simulink model "AmplifyFilterDryElectrodesCM"  (R2020b)
settings: Solver=VariableStepAuto  StartTime=0.0  StopTime=27  RelTol=1e-3
libraries: fl_lib x49, ee_lib x11, nesl_utility x6, simulink x2
settings Model: Creator=Miodrag Bolic  LastModifiedBy=bolic

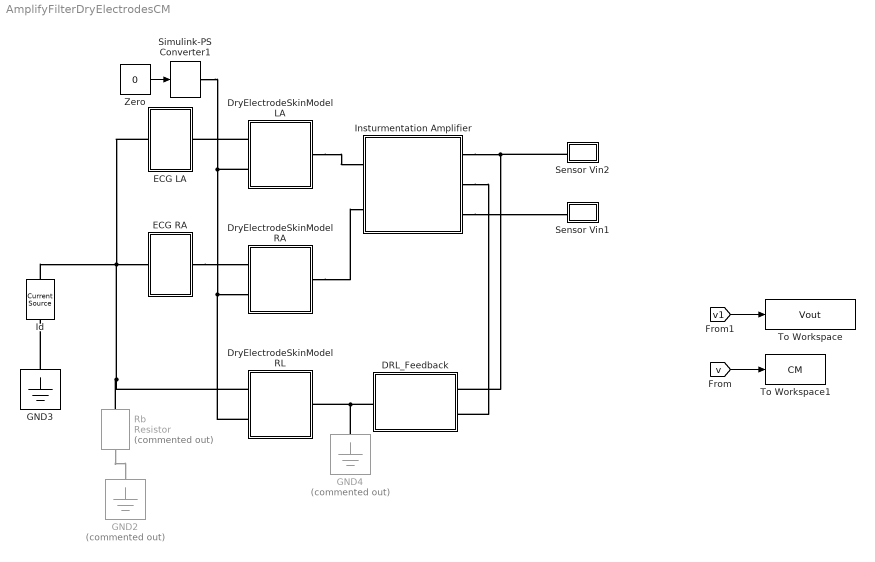
== system AmplifyFilterDryElectrodesCM ==
  DRL_Feedback : Subsystem
  DryElectrodeSkinModelLA : Subsystem
  DryElectrodeSkinModelRA : Subsystem
  DryElectrodeSkinModelRL : Subsystem
  ECG LA : Subsystem
  ECG RA : Subsystem
  GND2 : fl_lib/Electrical/Electrical Elements/Electrical Reference  Commented=on
  GND3 : fl_lib/Electrical/Electrical Elements/Electrical Reference
  GND4 : fl_lib/Electrical/Electrical Elements/Electrical Reference  Commented=on
  Id : ee_lib/Sources/Current Source  dc_current=0.2 uA  ac_current=0.2 uA  ac_shift=0 rad  ac_frequency=60 Hz  noise_mode=0  PSD=0 A^2/Hz  repeatability=1  auto_seed=113289902  user_seed=0  sample_time=1e-3 s  i_specify=off  i_priority=None  i=0 A  i_nominal_specify=off  i_nominal_unit=A  i_nominal_value=1  v_specify=off  v_priority=None  v=0 V  v_nominal_specify=off  v_nominal_unit=V  v_nominal_value=1
      settings: SourceProductBaseCode=PS
  Insturmentation Amplifier : Subsystem
  Rb : fl_lib/Electrical/Electrical Elements/Resistor  Commented=on  R=100 kOhm  i_specify=off  i_priority=None  i=0 A  i_nominal_specify=off  i_nominal_unit=A  i_nominal_value=1  v_specify=off  v_priority=None  v=0 V  v_nominal_specify=off  v_nominal_unit=V  v_nominal_value=1
      settings: AttributesFormatString=%<R> %<R_unit>
  Sensor Vin1 : Subsystem
      settings: PortSchema="{\"entries\":[{\"content\":{\"sides\":[{\"content\":{\"connectorIds\":[]},\"type\":\"ConnectorPlacement.EquallySpacedRectSide\",\"uuid\":\"3b18d6b5-859b-4059-8572-5738db8b00cf\"},{\"content\":{\"connectorIds\":[],\"side\":\"RIGHT\"},\"type\":\"ConnectorPlacement.EquallySpacedRectSide\",\"uuid\":\"93e2e2ec-1b37-410a-8244-321668873902\"},{\"content\":{\"connectorIds\":[\"LConn1\"],\"side\":\"TOP\"},\"type\":\"ConnectorPlacement.EquallySpacedRectSide\",\"uuid\":\"21d66db3-fc32-4ff6-a55a-49d3446fc8c3\"},{\"content\":{\"connectorIds\":[],\"side\":\"HIDDEN\"},\"type\":\"ConnectorPlacement.EquallySpacedRectSide\",\"uuid\":\"b4170d37-45a2-4670-be7d-b800aa089dd8\"}]},\"type\":\"ConnectorPlacement.EquallySpacedConnector\",\"uuid\":\"fdc20829-a084-458c-a3be-33b0b3d06234\"}],\"packageUris\":[\"http://schema.mathworks.com/mf0/Connector/R2020b\"],\"version\":\"1.0\"}"
      mask Display: disp('Vo')
  Sensor Vin2 : Subsystem
      settings: PortSchema="{\"entries\":[{\"content\":{\"sides\":[{\"content\":{\"connectorIds\":[]},\"type\":\"ConnectorPlacement.EquallySpacedRectSide\",\"uuid\":\"3b18d6b5-859b-4059-8572-5738db8b00cf\"},{\"content\":{\"connectorIds\":[],\"side\":\"RIGHT\"},\"type\":\"ConnectorPlacement.EquallySpacedRectSide\",\"uuid\":\"93e2e2ec-1b37-410a-8244-321668873902\"},{\"content\":{\"connectorIds\":[\"LConn1\"],\"side\":\"TOP\"},\"type\":\"ConnectorPlacement.EquallySpacedRectSide\",\"uuid\":\"21d66db3-fc32-4ff6-a55a-49d3446fc8c3\"},{\"content\":{\"connectorIds\":[],\"side\":\"HIDDEN\"},\"type\":\"ConnectorPlacement.EquallySpacedRectSide\",\"uuid\":\"b4170d37-45a2-4670-be7d-b800aa089dd8\"}]},\"type\":\"ConnectorPlacement.EquallySpacedConnector\",\"uuid\":\"fdc20829-a084-458c-a3be-33b0b3d06234\"}],\"packageUris\":[\"http://schema.mathworks.com/mf0/Connector/R2020b\"],\"version\":\"1.0\"}"
      mask Display: disp('Vcm')
  Simulink-PS Converter1 : nesl_utility/Simulink-PS Converter  PhysicalDomain=network_engine_domain  SubClassName=ps_input  LeftPortType=input  RightPortType=output  PseudoPeriodic=off  Frequencies=[]  NoiseDistribution=none  NoiseParameters=[]  Unit=1  AffineConversion=off  FilteringAndDerivatives=zero  SimscapeFilterOrder=1  InputFilterTimeConstant=0.001  UdotUserProvided=1
  To Workspace : ToWorkspace  VariableName=Vout  SaveFormat=Timeseries  SampleTime=-1
  To Workspace1 : ToWorkspace  VariableName=CM  SaveFormat=Timeseries  SampleTime=-1
  Zero : Constant  Value=0  OutDataTypeStr=Inherit: Inherit via back propagation
  wires:
  Zero/1 -> Simulink-PS Converter1/1
  [v] -> To Workspace1/1
  [v1] -> To Workspace/1
  connections:
  DryElectrodeSkinModelLA/LConn1 -- ECG LA/LConn1
  ECG LA/RConn1 -- DryElectrodeSkinModelRL/LConn1 -- Rb/LConn1 -- Id/LConn1 -- ECG RA/LConn1
  DryElectrodeSkinModelRA/RConn1 -- Insturmentation Amplifier/RConn2
  Simulink-PS Converter1/RConn1 -- DryElectrodeSkinModelLA/LConn2 -- DryElectrodeSkinModelRL/LConn2 -- DryElectrodeSkinModelRA/LConn2
  DryElectrodeSkinModelLA/RConn1 -- Insturmentation Amplifier/RConn1
  ECG RA/RConn1 -- DryElectrodeSkinModelRA/LConn1
  Rb/RConn1 -- GND2/LConn1
  Insturmentation Amplifier/LConn1 -- DRL_Feedback/RConn1 -- Sensor Vin2/LConn1
  Insturmentation Amplifier/LConn2 -- DRL_Feedback/RConn2
  GND3/LConn1 -- Id/RConn1
  DRL_Feedback/LConn1 -- GND4/LConn1 -- DryElectrodeSkinModelRL/RConn1
  Insturmentation Amplifier/LConn3 -- Sensor Vin1/LConn1

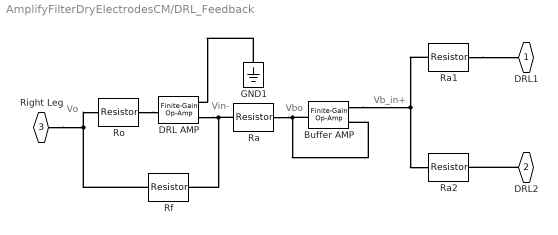
== system AmplifyFilterDryElectrodesCM/DRL_Feedback ==
  note: Vb_in+
  note: Vbo
  note: Vo
  note: Vin-
  Buffer AMP : ee_lib/Integrated Circuits/Finite-Gain Op-Amp  A=1000  Rin=1e+6 Ohm  Rout=100 Ohm  Vmin=-5 V  Vmax=5 V  noise_mode=0  v_noise=30e-9 V/Hz^0.50000  noise_prm=1  i_noise=0.5e-12 A/Hz^0.50000  ip_noise=0.5e-12 A/Hz^0.50000  in_noise=0.5e-12 A/Hz^0.50000  sample_time=1e-3 s  repeatability=1  auto_seed_v=1741257970  auto_seed_ip=3079639401  auto_seed_in=561050727  user_seed_v=0  user_seed_ip=0  user_seed_in=0
      settings: SourceProductBaseCode=PS  InternalSimscapePortConfiguration="{\"Bottom\":[],\"Left\":[{\"id\":\"p\",\"label\":\"+\",\"type\":\"foundation.electrical.electrical\"},{\"id\":\"n\",\"label\":\"-\",\"type\":\"foundation.electrical.electrical\"}],\"Right\":[{\"id\":\"out\",\"label\":\"\",\"type\":\"foundation.electrical.electrical\"}],\"Top\":[]}"
  DRL AMP : ee_lib/Integrated Circuits/Finite-Gain Op-Amp  A=1000  Rin=1e+6 Ohm  Rout=100 Ohm  Vmin=-5 V  Vmax=5 V  noise_mode=0  v_noise=30e-9 V/Hz^0.50000  noise_prm=1  i_noise=0.5e-12 A/Hz^0.50000  ip_noise=0.5e-12 A/Hz^0.50000  in_noise=0.5e-12 A/Hz^0.50000  sample_time=1e-3 s  repeatability=1  auto_seed_v=2070351588  auto_seed_ip=3106953985  auto_seed_in=1982177162  user_seed_v=0  user_seed_ip=0  user_seed_in=0
      settings: SourceProductBaseCode=PS  InternalSimscapePortConfiguration="{\"Bottom\":[],\"Left\":[{\"id\":\"p\",\"label\":\"+\",\"type\":\"foundation.electrical.electrical\"},{\"id\":\"n\",\"label\":\"-\",\"type\":\"foundation.electrical.electrical\"}],\"Right\":[{\"id\":\"out\",\"label\":\"\",\"type\":\"foundation.electrical.electrical\"}],\"Top\":[]}"
  GND1 : fl_lib/Electrical/Electrical Elements/Electrical Reference
  Ra : fl_lib/Electrical/Electrical Elements/Resistor  R=25 kOhm  i_specify=off  i_priority=None  i=0 A  i_nominal_specify=off  i_nominal_unit=A  i_nominal_value=1  v_specify=off  v_priority=None  v=0 V  v_nominal_specify=off  v_nominal_unit=V  v_nominal_value=1
      settings: AttributesFormatString=%<R> %<R_unit>
  Ra1 : fl_lib/Electrical/Electrical Elements/Resistor  R=25 kOhm  i_specify=off  i_priority=None  i=0 A  i_nominal_specify=off  i_nominal_unit=A  i_nominal_value=1  v_specify=off  v_priority=None  v=0 V  v_nominal_specify=off  v_nominal_unit=V  v_nominal_value=1
      settings: AttributesFormatString=%<R> %<R_unit>
  Ra2 : fl_lib/Electrical/Electrical Elements/Resistor  R=25 kOhm  i_specify=off  i_priority=None  i=0 A  i_nominal_specify=off  i_nominal_unit=A  i_nominal_value=1  v_specify=off  v_priority=None  v=0 V  v_nominal_specify=off  v_nominal_unit=V  v_nominal_value=1
      settings: AttributesFormatString=%<R> %<R_unit>
  Rf : fl_lib/Electrical/Electrical Elements/Resistor  R=2 MOhm  i_specify=off  i_priority=None  i=0 A  i_nominal_specify=off  i_nominal_unit=A  i_nominal_value=1  v_specify=off  v_priority=None  v=0 V  v_nominal_specify=off  v_nominal_unit=V  v_nominal_value=1
      settings: AttributesFormatString=%<R> %<R_unit>
  Ro : fl_lib/Electrical/Electrical Elements/Resistor  R=5 MOhm  i_specify=off  i_priority=None  i=0 A  i_nominal_specify=off  i_nominal_unit=A  i_nominal_value=1  v_specify=off  v_priority=None  v=0 V  v_nominal_specify=off  v_nominal_unit=V  v_nominal_value=1
      settings: AttributesFormatString=%<R> %<R_unit>
  DRL1 : PMIOPort  Side=Right
  DRL2 : PMIOPort  Port=2  Side=Right
  Right Leg : PMIOPort  Port=3  Side=Left
  connections:
  DRL2/RConn1 -- Ra2/RConn1
  Ra1/RConn1 -- DRL1/RConn1
  Ra1/LConn1 -- Buffer AMP/LConn1 -- Ra2/LConn1
  Ro/RConn1 -- DRL AMP/RConn1
  GND1/LConn1 -- DRL AMP/LConn1
  Rf/LConn1 -- Right Leg/RConn1 -- Ro/LConn1
  DRL AMP/LConn2 -- Ra/LConn1 -- Rf/RConn1
  Buffer AMP/RConn1 -- Ra/RConn1 -- Buffer AMP/LConn2

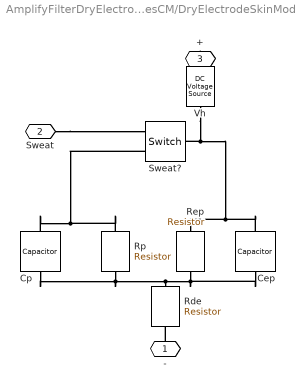
== system AmplifyFilterDryElectrodesCM/DryElectrodeSkinModelLA ==
  Cep : fl_lib/Electrical/Electrical Elements/Capacitor  c=10 nF  r=1e-6 Ohm  g=0 1/Ohm  i_specify=off  i_priority=None  i=0 A  i_nominal_specify=off  i_nominal_unit=A  i_nominal_value=1  v_specify=off  v_priority=None  v=0 V  v_nominal_specify=off  v_nominal_unit=V  v_nominal_value=1  vc_specify=on  vc_priority=High  vc=0 V  vc_nominal_specify=off  vc_nominal_unit=V  vc_nominal_value=1
      settings: AttributesFormatString=%<c> %<c_unit>
  Cp : fl_lib/Electrical/Electrical Elements/Capacitor  c=5 nF  r=1e-6 Ohm  g=0 1/Ohm  i_specify=off  i_priority=None  i=0 A  i_nominal_specify=off  i_nominal_unit=A  i_nominal_value=1  v_specify=off  v_priority=None  v=0 V  v_nominal_specify=off  v_nominal_unit=V  v_nominal_value=1  vc_specify=on  vc_priority=High  vc=0 V  vc_nominal_specify=off  vc_nominal_unit=V  vc_nominal_value=1
      settings: AttributesFormatString=%<c> %<c_unit>
  Rde : fl_lib/Electrical/Electrical Elements/Resistor  R=1 kOhm  i_specify=off  i_priority=None  i=0 A  i_nominal_specify=off  i_nominal_unit=A  i_nominal_value=1  v_specify=off  v_priority=None  v=0 V  v_nominal_specify=off  v_nominal_unit=V  v_nominal_value=1
  Rep : fl_lib/Electrical/Electrical Elements/Resistor  R=1 MOhm  i_specify=off  i_priority=None  i=0 A  i_nominal_specify=off  i_nominal_unit=A  i_nominal_value=1  v_specify=off  v_priority=None  v=0 V  v_nominal_specify=off  v_nominal_unit=V  v_nominal_value=1
      settings: AttributesFormatString=%<R> %<R_unit>
  Rp : fl_lib/Electrical/Electrical Elements/Resistor  R=10 kOhm  i_specify=off  i_priority=None  i=0 A  i_nominal_specify=off  i_nominal_unit=A  i_nominal_value=1  v_specify=off  v_priority=None  v=0 V  v_nominal_specify=off  v_nominal_unit=V  v_nominal_value=1
      settings: AttributesFormatString=%<R> %<R_unit>
  Sweat? : fl_lib/Electrical/Electrical Elements/Switch  R_closed=0.01 Ohm  G_open=1e-8 1/Ohm  Threshold=0.5  i_specify=off  i_priority=None  i=0 A  i_nominal_specify=off  i_nominal_unit=A  i_nominal_value=1  v_specify=off  v_priority=None  v=0 V  v_nominal_specify=off  v_nominal_unit=V  v_nominal_value=1
  Vh : fl_lib/Electrical/Electrical Sources/DC Voltage Source  v0=230 mV
      settings: AttributesFormatString=%<v0> %<v0_unit>
  - : PMIOPort  Side=Left
  Sweat : PMIOPort  Port=2  Side=Left
  + : PMIOPort  Port=3  Side=Right
  connections:
  Rp/RConn1 -- Sweat?/RConn2 -- Cp/RConn1
  Vh/LConn1 -- +/RConn1
  Sweat/RConn1 -- Sweat?/RConn1
  Sweat?/LConn1 -- Cep/RConn1 -- Rep/RConn1 -- Vh/RConn1
  Rp/LConn1 -- Cp/LConn1 -- Cep/LConn1 -- Rep/LConn1 -- Rde/LConn1
  -/RConn1 -- Rde/RConn1

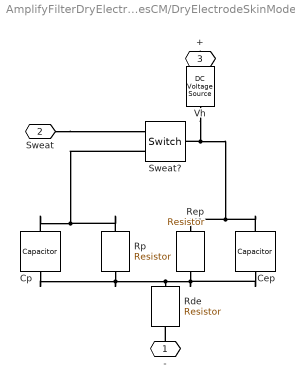
== system AmplifyFilterDryElectrodesCM/DryElectrodeSkinModelRA ==
  Cep : fl_lib/Electrical/Electrical Elements/Capacitor  c=10 nF  r=1e-6 Ohm  g=0 1/Ohm  i_specify=off  i_priority=None  i=0 A  i_nominal_specify=off  i_nominal_unit=A  i_nominal_value=1  v_specify=off  v_priority=None  v=0 V  v_nominal_specify=off  v_nominal_unit=V  v_nominal_value=1  vc_specify=on  vc_priority=High  vc=0 V  vc_nominal_specify=off  vc_nominal_unit=V  vc_nominal_value=1
      settings: AttributesFormatString=%<c> %<c_unit>
  Cp : fl_lib/Electrical/Electrical Elements/Capacitor  c=5 nF  r=1e-6 Ohm  g=0 1/Ohm  i_specify=off  i_priority=None  i=0 A  i_nominal_specify=off  i_nominal_unit=A  i_nominal_value=1  v_specify=off  v_priority=None  v=0 V  v_nominal_specify=off  v_nominal_unit=V  v_nominal_value=1  vc_specify=on  vc_priority=High  vc=0 V  vc_nominal_specify=off  vc_nominal_unit=V  vc_nominal_value=1
      settings: AttributesFormatString=%<c> %<c_unit>
  Rde : fl_lib/Electrical/Electrical Elements/Resistor  R=1 kOhm  i_specify=off  i_priority=None  i=0 A  i_nominal_specify=off  i_nominal_unit=A  i_nominal_value=1  v_specify=off  v_priority=None  v=0 V  v_nominal_specify=off  v_nominal_unit=V  v_nominal_value=1
  Rep : fl_lib/Electrical/Electrical Elements/Resistor  R=1 MOhm  i_specify=off  i_priority=None  i=0 A  i_nominal_specify=off  i_nominal_unit=A  i_nominal_value=1  v_specify=off  v_priority=None  v=0 V  v_nominal_specify=off  v_nominal_unit=V  v_nominal_value=1
      settings: AttributesFormatString=%<R> %<R_unit>
  Rp : fl_lib/Electrical/Electrical Elements/Resistor  R=10 kOhm  i_specify=off  i_priority=None  i=0 A  i_nominal_specify=off  i_nominal_unit=A  i_nominal_value=1  v_specify=off  v_priority=None  v=0 V  v_nominal_specify=off  v_nominal_unit=V  v_nominal_value=1
      settings: AttributesFormatString=%<R> %<R_unit>
  Sweat? : fl_lib/Electrical/Electrical Elements/Switch  R_closed=0.01 Ohm  G_open=1e-8 1/Ohm  Threshold=0.5  i_specify=off  i_priority=None  i=0 A  i_nominal_specify=off  i_nominal_unit=A  i_nominal_value=1  v_specify=off  v_priority=None  v=0 V  v_nominal_specify=off  v_nominal_unit=V  v_nominal_value=1
  Vh : fl_lib/Electrical/Electrical Sources/DC Voltage Source  v0=230 mV
      settings: AttributesFormatString=%<v0> %<v0_unit>
  - : PMIOPort  Side=Left
  Sweat : PMIOPort  Port=2  Side=Left
  + : PMIOPort  Port=3  Side=Right
  connections:
  Rp/RConn1 -- Sweat?/RConn2 -- Cp/RConn1
  Vh/LConn1 -- +/RConn1
  Sweat/RConn1 -- Sweat?/RConn1
  Sweat?/LConn1 -- Cep/RConn1 -- Rep/RConn1 -- Vh/RConn1
  Cp/LConn1 -- Rp/LConn1 -- Cep/LConn1 -- Rep/LConn1 -- Rde/LConn1
  -/RConn1 -- Rde/RConn1

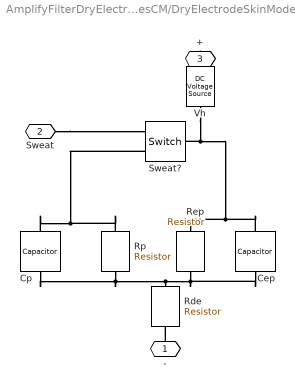
== system AmplifyFilterDryElectrodesCM/DryElectrodeSkinModelRL ==
  Cep : fl_lib/Electrical/Electrical Elements/Capacitor  c=10 nF  r=1e-6 Ohm  g=0 1/Ohm  i_specify=off  i_priority=None  i=0 A  i_nominal_specify=off  i_nominal_unit=A  i_nominal_value=1  v_specify=off  v_priority=None  v=0 V  v_nominal_specify=off  v_nominal_unit=V  v_nominal_value=1  vc_specify=on  vc_priority=High  vc=0 V  vc_nominal_specify=off  vc_nominal_unit=V  vc_nominal_value=1
      settings: AttributesFormatString=%<c> %<c_unit>
  Cp : fl_lib/Electrical/Electrical Elements/Capacitor  c=5 nF  r=1e-6 Ohm  g=0 1/Ohm  i_specify=off  i_priority=None  i=0 A  i_nominal_specify=off  i_nominal_unit=A  i_nominal_value=1  v_specify=off  v_priority=None  v=0 V  v_nominal_specify=off  v_nominal_unit=V  v_nominal_value=1  vc_specify=on  vc_priority=High  vc=0 V  vc_nominal_specify=off  vc_nominal_unit=V  vc_nominal_value=1
      settings: AttributesFormatString=%<c> %<c_unit>
  Rde : fl_lib/Electrical/Electrical Elements/Resistor  R=1 kOhm  i_specify=off  i_priority=None  i=0 A  i_nominal_specify=off  i_nominal_unit=A  i_nominal_value=1  v_specify=off  v_priority=None  v=0 V  v_nominal_specify=off  v_nominal_unit=V  v_nominal_value=1
      settings: AttributesFormatString=|
      | %<R>
      | %<R_unit>
  Rep : fl_lib/Electrical/Electrical Elements/Resistor  R=1 MOhm  i_specify=off  i_priority=None  i=0 A  i_nominal_specify=off  i_nominal_unit=A  i_nominal_value=1  v_specify=off  v_priority=None  v=0 V  v_nominal_specify=off  v_nominal_unit=V  v_nominal_value=1
      settings: AttributesFormatString=%<R> %<R_unit>
  Rp : fl_lib/Electrical/Electrical Elements/Resistor  R=10 kOhm  i_specify=off  i_priority=None  i=0 A  i_nominal_specify=off  i_nominal_unit=A  i_nominal_value=1  v_specify=off  v_priority=None  v=0 V  v_nominal_specify=off  v_nominal_unit=V  v_nominal_value=1
      settings: AttributesFormatString=%<R> %<R_unit>
  Sweat? : fl_lib/Electrical/Electrical Elements/Switch  R_closed=0.01 Ohm  G_open=1e-8 1/Ohm  Threshold=0.5  i_specify=off  i_priority=None  i=0 A  i_nominal_specify=off  i_nominal_unit=A  i_nominal_value=1  v_specify=off  v_priority=None  v=0 V  v_nominal_specify=off  v_nominal_unit=V  v_nominal_value=1
  Vh : fl_lib/Electrical/Electrical Sources/DC Voltage Source  v0=230 mV
      settings: AttributesFormatString=%<v0> %<v0_unit>
  - : PMIOPort  Side=Left
  Sweat : PMIOPort  Port=2  Side=Left
  + : PMIOPort  Port=3  Side=Right
  connections:
  Rp/RConn1 -- Sweat?/RConn2 -- Cp/RConn1
  Vh/LConn1 -- +/RConn1
  Sweat/RConn1 -- Sweat?/RConn1
  Sweat?/LConn1 -- Cep/RConn1 -- Rep/RConn1 -- Vh/RConn1
  Cp/LConn1 -- Rp/LConn1 -- Cep/LConn1 -- Rep/LConn1 -- Rde/LConn1
  -/RConn1 -- Rde/RConn1

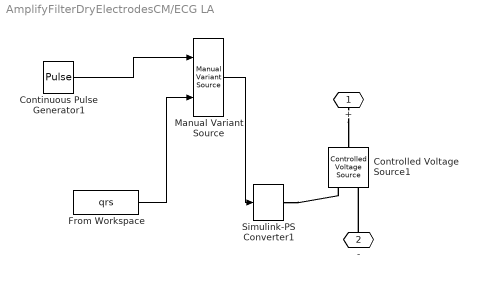
== system AmplifyFilterDryElectrodesCM/ECG LA ==
  Continuous Pulse Generator1 : DiscretePulseGenerator  PulseType=Time based  Amplitude=0.001  Period=1  PulseWidth=10
  Controlled Voltage Source1 : fl_lib/Electrical/Electrical Sources/Controlled Voltage Source
  From Workspace : FromWorkspace  VariableName=qrs  SampleTime=0.004  OutputAfterFinalValue=Setting to zero
  Manual Variant Source : simulink/Signal Routing/Manual Variant Source  NumChoices=2  LabelModeActiveChoice=V_2
  Simulink-PS Converter1 : nesl_utility/Simulink-PS Converter  PhysicalDomain=network_engine_domain  SubClassName=ps_input  LeftPortType=input  RightPortType=output  PseudoPeriodic=off  Frequencies=[]  NoiseDistribution=none  NoiseParameters=[]  Unit=1  AffineConversion=off  FilteringAndDerivatives=zero  SimscapeFilterOrder=1  InputFilterTimeConstant=0.001  UdotUserProvided=1
  + : PMIOPort  Side=Left
  - : PMIOPort  Port=2  Side=Right
  wires:
  From Workspace/1 -> Manual Variant Source/2
  Manual Variant Source/1 -> Simulink-PS Converter1/1
  Continuous Pulse Generator1/1 -> Manual Variant Source/1
  connections:
  Simulink-PS Converter1/RConn1 -- Controlled Voltage Source1/RConn1
  +/RConn1 -- Controlled Voltage Source1/LConn1
  -/RConn1 -- Controlled Voltage Source1/RConn2

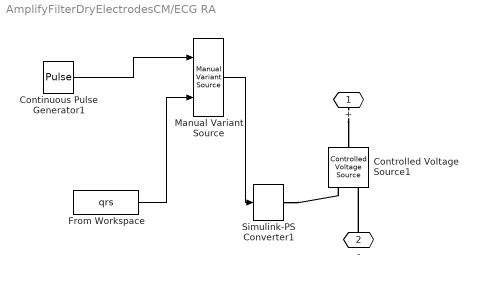
== system AmplifyFilterDryElectrodesCM/ECG RA ==
  Continuous Pulse Generator1 : DiscretePulseGenerator  PulseType=Time based  Amplitude=0.001  Period=1  PulseWidth=10
  Controlled Voltage Source1 : fl_lib/Electrical/Electrical Sources/Controlled Voltage Source
  From Workspace : FromWorkspace  VariableName=qrs  SampleTime=0.004  OutputAfterFinalValue=Setting to zero
  Manual Variant Source : simulink/Signal Routing/Manual Variant Source  NumChoices=2  LabelModeActiveChoice=V_2
  Simulink-PS Converter1 : nesl_utility/Simulink-PS Converter  PhysicalDomain=network_engine_domain  SubClassName=ps_input  LeftPortType=input  RightPortType=output  PseudoPeriodic=off  Frequencies=[]  NoiseDistribution=none  NoiseParameters=[]  Unit=1  AffineConversion=off  FilteringAndDerivatives=zero  SimscapeFilterOrder=1  InputFilterTimeConstant=0.001  UdotUserProvided=1
  + : PMIOPort  Side=Left
  - : PMIOPort  Port=2  Side=Right
  wires:
  From Workspace/1 -> Manual Variant Source/2
  Manual Variant Source/1 -> Simulink-PS Converter1/1
  Continuous Pulse Generator1/1 -> Manual Variant Source/1
  connections:
  Simulink-PS Converter1/RConn1 -- Controlled Voltage Source1/RConn1
  +/RConn1 -- Controlled Voltage Source1/LConn1
  -/RConn1 -- Controlled Voltage Source1/RConn2

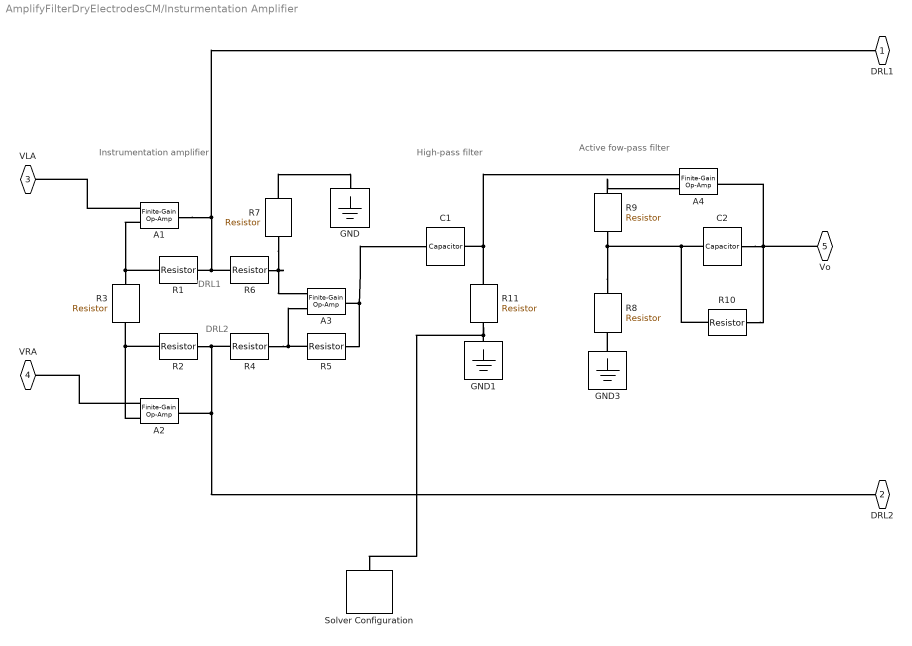
== system AmplifyFilterDryElectrodesCM/Insturmentation Amplifier ==
  note: Active fow-pass filter
  note: High-pass filter
  note: DRL2
  note: Instrumentation amplifier
  note: DRL1
  A1 : ee_lib/Integrated Circuits/Finite-Gain Op-Amp  A=10000  Rin=1e+8 Ohm  Rout=100 Ohm  Vmin=-5 V  Vmax=5 V  noise_mode=0  v_noise=30e-9 V/Hz^0.50000  noise_prm=1  i_noise=0.5e-12 A/Hz^0.50000  ip_noise=0.5e-12 A/Hz^0.50000  in_noise=0.5e-12 A/Hz^0.50000  sample_time=1e-3 s  repeatability=1  auto_seed_v=1146474661  auto_seed_ip=3669999592  auto_seed_in=3134143196  user_seed_v=0  user_seed_ip=0  user_seed_in=0
      settings: SourceProductBaseCode=PS  InternalSimscapePortConfiguration="{\"Bottom\":[],\"Left\":[{\"id\":\"p\",\"label\":\"+\",\"type\":\"foundation.electrical.electrical\"},{\"id\":\"n\",\"label\":\"-\",\"type\":\"foundation.electrical.electrical\"}],\"Right\":[{\"id\":\"out\",\"label\":\"\",\"type\":\"foundation.electrical.electrical\"}],\"Top\":[]}"
  A2 : ee_lib/Integrated Circuits/Finite-Gain Op-Amp  A=10000  Rin=1e+8 Ohm  Rout=100 Ohm  Vmin=-5 V  Vmax=5 V  noise_mode=0  v_noise=30e-9 V/Hz^0.50000  noise_prm=1  i_noise=0.5e-12 A/Hz^0.50000  ip_noise=0.5e-12 A/Hz^0.50000  in_noise=0.5e-12 A/Hz^0.50000  sample_time=1e-3 s  repeatability=1  auto_seed_v=1055092266  auto_seed_ip=2954699273  auto_seed_in=1182424479  user_seed_v=0  user_seed_ip=0  user_seed_in=0
      settings: SourceProductBaseCode=PS  InternalSimscapePortConfiguration="{\"Bottom\":[],\"Left\":[{\"id\":\"p\",\"label\":\"+\",\"type\":\"foundation.electrical.electrical\"},{\"id\":\"n\",\"label\":\"-\",\"type\":\"foundation.electrical.electrical\"}],\"Right\":[{\"id\":\"out\",\"label\":\"\",\"type\":\"foundation.electrical.electrical\"}],\"Top\":[]}"
  A3 : ee_lib/Integrated Circuits/Finite-Gain Op-Amp  A=1000  Rin=1e+6 Ohm  Rout=100 Ohm  Vmin=-5 V  Vmax=5 V  noise_mode=0  v_noise=30e-9 V/Hz^0.50000  noise_prm=1  i_noise=0.5e-12 A/Hz^0.50000  ip_noise=0.5e-12 A/Hz^0.50000  in_noise=0.5e-12 A/Hz^0.50000  sample_time=1e-3 s  repeatability=1  auto_seed_v=2730578035  auto_seed_ip=313293061  auto_seed_in=4055586805  user_seed_v=0  user_seed_ip=0  user_seed_in=0
      settings: SourceProductBaseCode=PS  InternalSimscapePortConfiguration="{\"Bottom\":[],\"Left\":[{\"id\":\"p\",\"label\":\"+\",\"type\":\"foundation.electrical.electrical\"},{\"id\":\"n\",\"label\":\"-\",\"type\":\"foundation.electrical.electrical\"}],\"Right\":[{\"id\":\"out\",\"label\":\"\",\"type\":\"foundation.electrical.electrical\"}],\"Top\":[]}"
  A4 : ee_lib/Integrated Circuits/Finite-Gain Op-Amp  A=1000  Rin=1e+6 Ohm  Rout=100 Ohm  Vmin=-5 V  Vmax=5 V  noise_mode=0  v_noise=30e-9 V/Hz^0.50000  noise_prm=1  i_noise=0.5e-12 A/Hz^0.50000  ip_noise=0.5e-12 A/Hz^0.50000  in_noise=0.5e-12 A/Hz^0.50000  sample_time=1e-3 s  repeatability=1  auto_seed_v=476463885  auto_seed_ip=107962283  auto_seed_in=2557701871  user_seed_v=0  user_seed_ip=0  user_seed_in=0
      settings: SourceProductBaseCode=PS  InternalSimscapePortConfiguration="{\"Bottom\":[],\"Left\":[{\"id\":\"p\",\"label\":\"+\",\"type\":\"foundation.electrical.electrical\"},{\"id\":\"n\",\"label\":\"-\",\"type\":\"foundation.electrical.electrical\"}],\"Right\":[{\"id\":\"out\",\"label\":\"\",\"type\":\"foundation.electrical.electrical\"}],\"Top\":[]}"
  C1 : fl_lib/Electrical/Electrical Elements/Capacitor  c=1 uF  r=1e-6 Ohm  g=0 1/Ohm  i_specify=off  i_priority=None  i=0 A  i_nominal_specify=off  i_nominal_unit=A  i_nominal_value=1  v_specify=off  v_priority=None  v=0 V  v_nominal_specify=off  v_nominal_unit=V  v_nominal_value=1  vc_specify=on  vc_priority=High  vc=0 V  vc_nominal_specify=off  vc_nominal_unit=V  vc_nominal_value=1
      settings: AttributesFormatString=%<c> %<c_unit>
  C2 : fl_lib/Electrical/Electrical Elements/Capacitor  c=0.01 uF  r=1e-6 Ohm  g=0 1/Ohm  i_specify=off  i_priority=None  i=0 A  i_nominal_specify=off  i_nominal_unit=A  i_nominal_value=1  v_specify=off  v_priority=None  v=0 V  v_nominal_specify=off  v_nominal_unit=V  v_nominal_value=1  vc_specify=on  vc_priority=High  vc=0 V  vc_nominal_specify=off  vc_nominal_unit=V  vc_nominal_value=1
      settings: AttributesFormatString=%<c> %<c_unit>
  GND : fl_lib/Electrical/Electrical Elements/Electrical Reference
  GND1 : fl_lib/Electrical/Electrical Elements/Electrical Reference
  GND3 : fl_lib/Electrical/Electrical Elements/Electrical Reference
  R1 : fl_lib/Electrical/Electrical Elements/Resistor  R=25 kOhm  i_specify=off  i_priority=None  i=0 A  i_nominal_specify=off  i_nominal_unit=A  i_nominal_value=1  v_specify=off  v_priority=None  v=0 V  v_nominal_specify=off  v_nominal_unit=V  v_nominal_value=1
      settings: AttributesFormatString=|
      | %<R>
      | %<R_unit>
  R10 : fl_lib/Electrical/Electrical Elements/Resistor  R=150 kOhm  i_specify=off  i_priority=None  i=0 A  i_nominal_specify=off  i_nominal_unit=A  i_nominal_value=1  v_specify=off  v_priority=None  v=0 V  v_nominal_specify=off  v_nominal_unit=V  v_nominal_value=1
      settings: AttributesFormatString=%<R> %<R_unit>
  R11 : fl_lib/Electrical/Electrical Elements/Resistor  R=3.2 MOhm  i_specify=off  i_priority=None  i=0 A  i_nominal_specify=off  i_nominal_unit=A  i_nominal_value=1  v_specify=off  v_priority=None  v=0 V  v_nominal_specify=off  v_nominal_unit=V  v_nominal_value=1
      settings: AttributesFormatString=%<R> %<R_unit>
  R2 : fl_lib/Electrical/Electrical Elements/Resistor  R=25 kOhm  i_specify=off  i_priority=None  i=0 A  i_nominal_specify=off  i_nominal_unit=A  i_nominal_value=1  v_specify=off  v_priority=None  v=0 V  v_nominal_specify=off  v_nominal_unit=V  v_nominal_value=1
      settings: AttributesFormatString=|
      | %<R>
      | %<R_unit>
  R3 : fl_lib/Electrical/Electrical Elements/Resistor  R=5.5 kOhm  i_specify=off  i_priority=None  i=0 A  i_nominal_specify=off  i_nominal_unit=A  i_nominal_value=1  v_specify=off  v_priority=None  v=0 V  v_nominal_specify=off  v_nominal_unit=V  v_nominal_value=1
      settings: AttributesFormatString=|
      | %<R>
      | %<R_unit>
  R4 : ee_lib/Passive/Resistor  R=25 kOhm  R_tol=1  enable_R_tol=2  tol_distribution=1  nSigma=4  enable_operating_limits=0  operating_limit_action=2  max_working_voltage=100 V  power_rating=1 W  enable_faults=0  fault_action=1  R_faulted=inf Ohm  enable_temporal_fault=0  t_fault=1 s  enable_behavioral_fault=0  max_permissible_current=1 A  t_fail_on_current=1 s  noise_mode=0  sample_time=1e-3 s  repeatability=1  auto_seed=2474664379  user_seed=0  Tdevice=25 degC  alpha=3.93e-3 1/K  Tmeas=25 degC  thermal_mass=100 J/K  power_derating_T1=70 degC  power_derating_T2=155 degC  operating_temperature_range_vec=[-50, 150] degC  temperature_specify=off  temperature_priority=High  temperature=298.15 K  temperature_nominal_specify=off  temperature_nominal_unit=K  temperature_nominal_value=1
      settings: AttributesFormatString=|
      | %<R>
      | %<R_unit>
  R5 : ee_lib/Passive/Resistor  R=25 kOhm  R_tol=1  enable_R_tol=3  tol_distribution=1  nSigma=4  enable_operating_limits=0  operating_limit_action=2  max_working_voltage=100 V  power_rating=1 W  enable_faults=0  fault_action=1  R_faulted=inf Ohm  enable_temporal_fault=0  t_fault=1 s  enable_behavioral_fault=0  max_permissible_current=1 A  t_fail_on_current=1 s  noise_mode=0  sample_time=1e-3 s  repeatability=1  auto_seed=1334967464  user_seed=0  Tdevice=25 degC  alpha=3.93e-3 1/K  Tmeas=25 degC  thermal_mass=100 J/K  power_derating_T1=70 degC  power_derating_T2=155 degC  operating_temperature_range_vec=[-50, 150] degC  temperature_specify=off  temperature_priority=High  temperature=298.15 K  temperature_nominal_specify=off  temperature_nominal_unit=K  temperature_nominal_value=1
      settings: AttributesFormatString=|
      | %<R>
      | %<R_unit>
  R6 : ee_lib/Passive/Resistor  R=25 kOhm  R_tol=1  enable_R_tol=3  tol_distribution=1  nSigma=4  enable_operating_limits=0  operating_limit_action=2  max_working_voltage=100 V  power_rating=1 W  enable_faults=0  fault_action=1  R_faulted=inf Ohm  enable_temporal_fault=0  t_fault=1 s  enable_behavioral_fault=0  max_permissible_current=1 A  t_fail_on_current=1 s  noise_mode=0  sample_time=1e-3 s  repeatability=1  auto_seed=4117119081  user_seed=0  Tdevice=25 degC  alpha=3.93e-3 1/K  Tmeas=25 degC  thermal_mass=100 J/K  power_derating_T1=70 degC  power_derating_T2=155 degC  operating_temperature_range_vec=[-50, 150] degC  temperature_specify=off  temperature_priority=High  temperature=298.15 K  temperature_nominal_specify=off  temperature_nominal_unit=K  temperature_nominal_value=1
      settings: AttributesFormatString=|
      | %<R>
      | %<R_unit>
  R7 : ee_lib/Passive/Resistor  R=25 kOhm  R_tol=1  enable_R_tol=2  tol_distribution=1  nSigma=4  enable_operating_limits=0  operating_limit_action=2  max_working_voltage=100 V  power_rating=1 W  enable_faults=0  fault_action=1  R_faulted=inf Ohm  enable_temporal_fault=0  t_fault=1 s  enable_behavioral_fault=0  max_permissible_current=1 A  t_fail_on_current=1 s  noise_mode=0  sample_time=1e-3 s  repeatability=1  auto_seed=2554089351  user_seed=0  Tdevice=25 degC  alpha=3.93e-3 1/K  Tmeas=25 degC  thermal_mass=100 J/K  power_derating_T1=70 degC  power_derating_T2=155 degC  operating_temperature_range_vec=[-50, 150] degC  temperature_specify=off  temperature_priority=High  temperature=298.15 K  temperature_nominal_specify=off  temperature_nominal_unit=K  temperature_nominal_value=1
      settings: AttributesFormatString=|
      | %<R>
      | %<R_unit>
  R8 : fl_lib/Electrical/Electrical Elements/Resistor  R=4.7 kOhm  i_specify=off  i_priority=None  i=0 A  i_nominal_specify=off  i_nominal_unit=A  i_nominal_value=1  v_specify=off  v_priority=None  v=0 V  v_nominal_specify=off  v_nominal_unit=V  v_nominal_value=1
      settings: AttributesFormatString=%<R> %<R_unit>
  R9 : fl_lib/Electrical/Electrical Elements/Resistor  R=3.3 MOhm  i_specify=off  i_priority=None  i=0 A  i_nominal_specify=off  i_nominal_unit=A  i_nominal_value=1  v_specify=off  v_priority=None  v=0 V  v_nominal_specify=off  v_nominal_unit=V  v_nominal_value=1
      settings: AttributesFormatString=%<R> %<R_unit>
  "Solver Configuration " : nesl_utility/Solver Configuration  PhysicalDomain=network_engine_domain  SubClassName=solver  LeftPortType=input  RightPortType=generic  Tones=[]  Harmonics=[]  SimulateNoise=off  Profile=off  UseLocalSampling=off  EnableSwitchedLinearOptims=on  FrequencyDomain=off  UseCCode=off  RelTol=0.001  AbsTol=1e-06  MinStep=1e-09  ToWorkspace=off  RevertToSquareIcSolve=off  NumHomotopyIterations=100  PhasorMode=off  PhasorModeNumHarmonics=1  DoDC=off  ResidualTolerance=1e-09  UseLocalSolver=on  LocalSolverChoice=NE_BACKWARD_EULER_ADVANCER  LocalSolverSampleTime=0.001  DoFixedCost=on  MaxNonlinIter=3  MaxModeIter=2  ComputeImpulses=off  ImpulseIterations=2  LinearAlgebra=Sparse  EquationFormulation=NE_TIME_EF  DelaysMemoryBudget=1024  AutomaticFiltering=on  FilteringTimeConstant=0.001  PartitionStorageMethod=AS_NEEDED  PartitionMemoryBudget=1024  PartitionMethod=FAST
  DRL1 : PMIOPort  Side=Left
  DRL2 : PMIOPort  Port=2  Side=Left
  VLA : PMIOPort  Port=3  Side=Right
  VRA : PMIOPort  Port=4  Side=Right
  Vo : PMIOPort  Port=5  Side=Left
  connections:
  R11/RConn1 -- "Solver Configuration "/RConn1 -- GND1/LConn1
  R8/LConn1 -- R10/LConn1 -- C2/LConn1 -- R9/RConn1
  C1/RConn1 -- R11/LConn1 -- A4/LConn1
  R10/RConn1 -- C2/RConn1 -- Vo/RConn1 -- A4/RConn1
  R9/LConn1 -- A4/LConn2
  GND3/LConn1 -- R8/RConn1
  R5/LConn1 -- A3/LConn2 -- R4/RConn1
  A2/LConn2 -- R2/LConn1 -- R3/RConn1
  A2/RConn1 -- DRL2/RConn1 -- R2/RConn1 -- R4/LConn1
  R6/RConn1 -- A3/LConn1 -- R7/LConn1
  R5/RConn1 -- C1/LConn1 -- A3/RConn1
  R1/RConn1 -- DRL1/RConn1 -- A1/RConn1 -- R6/LConn1
  R3/LConn1 -- R1/LConn1 -- A1/LConn2
  A1/LConn1 -- VLA/RConn1
  A2/LConn1 -- VRA/RConn1
  R7/RConn1 -- GND/LConn1

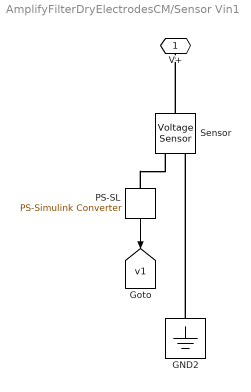
== system AmplifyFilterDryElectrodesCM/Sensor Vin1 ==
  GND2 : fl_lib/Electrical/Electrical Elements/Electrical Reference
  PS-SL : nesl_utility/PS-Simulink Converter  PhysicalDomain=network_engine_domain  SubClassName=ps_output  LeftPortType=input  RightPortType=output  PseudoPeriodic=off  Frequencies=[]  Unit=1  AffineConversion=off
  Sensor : fl_lib/Electrical/Electrical Sensors/Voltage Sensor
      settings: SourceProductName=Foundation Library
  V+ : PMIOPort  Side=Left
  tag scope: v1=global
  wires:
  PS-SL/1 -> [v1]
  connections:
  PS-SL/LConn1 -- Sensor/RConn1
  Sensor/LConn1 -- V+/RConn1
  GND2/LConn1 -- Sensor/RConn2

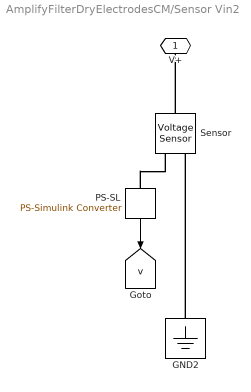
== system AmplifyFilterDryElectrodesCM/Sensor Vin2 ==
  GND2 : fl_lib/Electrical/Electrical Elements/Electrical Reference
  PS-SL : nesl_utility/PS-Simulink Converter  PhysicalDomain=network_engine_domain  SubClassName=ps_output  LeftPortType=input  RightPortType=output  PseudoPeriodic=off  Frequencies=[]  Unit=1  AffineConversion=off
  Sensor : fl_lib/Electrical/Electrical Sensors/Voltage Sensor
      settings: SourceProductName=Foundation Library
  V+ : PMIOPort  Side=Left
  tag scope: v=global
  wires:
  PS-SL/1 -> [v]
  connections:
  PS-SL/LConn1 -- Sensor/RConn1
  Sensor/LConn1 -- V+/RConn1
  GND2/LConn1 -- Sensor/RConn2
